simulink model "BLAC0_ControlloCoppiaCompensazioneFCEM"  (R2018b)
settings: Solver=VariableStepAuto  StartTime=0.0  StopTime=0.1  RelTol=1e-3
values from neighbouring files (symbols this model uses):
  B = 3.8e-005    (= 3.8e-05)    [BLAC0_v1.m]    (also in BLAC1_v1.m = 0; BLAC1_v2.m = 0; CAE_11_v_1.m = 0; CAE_14_v1.M = 0)
  Crn = 0.6    [BLAC0_v1.m]    (also in BLAC1_v1.m; BLAC1_v2.m; CAE_11_v_1.m; CAE_14_v1.M)
  J = 0.0000251    (= 2.51e-05)    [BLAC0_v1.m]    (also in BLAC1_v1.m = 0.001; BLAC1_v2.m = 0.001; CAE_11_v_1.m = 0.001; CAE_14_v1.M = 0.001)
  Kc = ms*np*lambdaf/2    (= 0.27)    [BLAC0_v1.m]    (also in BLAC1_v1.m = 0.6; BLAC1_v2.m = 0.6; CAE_11_v_1.m = 0.6; CAE_14_v1.M = 0.6)
  Lsd = 0.005/2    (= 0.0025)    [BLAC0_v1.m]    (also in BLAC1_v1.m = 0.005; BLAC1_v2.m = 0.005; CAE_11_v_1.m = 0.005; CAE_14_v1.M = 0.005)
  Lsq = Lsd    (= 0.0025)    [BLAC0_v1.m]    (also in BLAC1_v1.m = 0.005; BLAC1_v2.m = 0.005; CAE_11_v_1.m = 0.005; CAE_14_v1.M = 0.005)
  np = 2    [BLAC0_v1.m]    (also in BLAC1_v1.m = 4; BLAC1_v2.m = 4; CAE_11_v_1.m = 4; CAE_14_v1.M = 4)
  PSIPM = lambdaf    (= 0.09)    [BLAC0_v1.m]
  Rs = 3.1/2    (= 1.55)    [BLAC0_v1.m]    (also in BLAC1_v1.m = 1; BLAC1_v2.m = 1; CAE_11_v_1.m = 1; CAE_14_v1.M = 1)
  wrr = 1256.6    [BLAC0_v1.m]    (also in BLAC1_v1.m = 300; BLAC1_v2.m = 300)
settings Model: Creator=anton  LastModifiedBy=anton

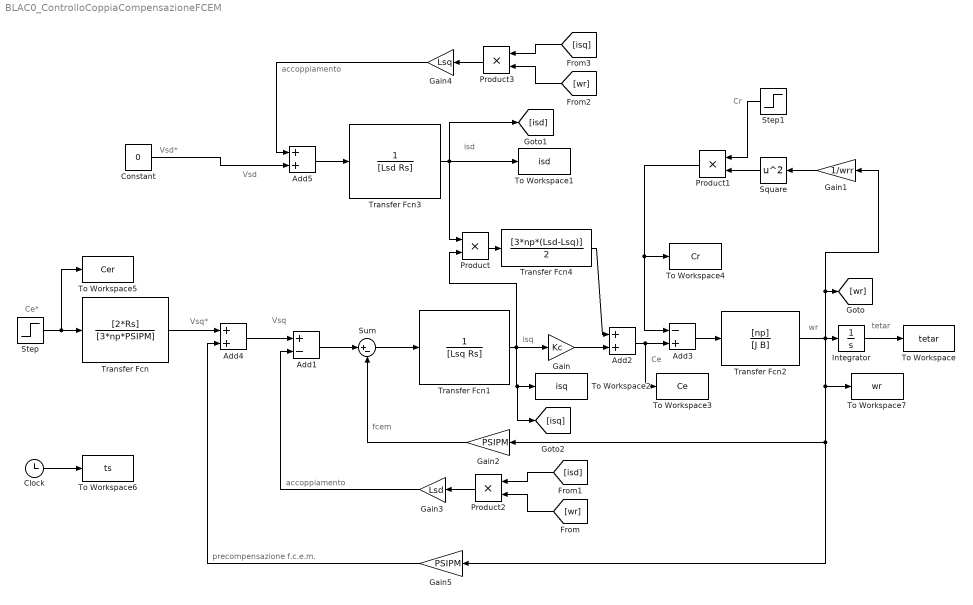
== system BLAC0_ControlloCoppiaCompensazioneFCEM ==
  note: precompensazione f.c.e.m.
  note: accoppiamento
  note: accoppiamento
  note: fcem
  note: Cr
  note: isd
  note: Vsd
  note: Vsd*
  note: tetar
  note: wr
  note: Ce
  note: isq
  note: Vsq
  note: Vsq*
  note: Ce*
  Add1 : Sum  Inputs=+-
  Add2 : Sum
  Add3 : Sum  Inputs=-+
  Add4 : Sum
  Add5 : Sum
  Clock : Clock
  Constant : Constant  Value=0
  Gain : Gain  Gain=Kc
  Gain1 : Gain  Gain=1/wrr
  Gain2 : Gain  Gain=PSIPM
  Gain3 : Gain  Gain=Lsd
  Gain4 : Gain  Gain=Lsq
  Gain5 : Gain  Gain=PSIPM
  Integrator : Integrator
  Product{,1..3} (4 alike) : Product
  Square : Math  Operator=square  SaturateOnIntegerOverflow=on
  Step : Step  Time=0  After=Crn  SampleTime=0
  Step1 : Step  Time=0  After=Crn  SampleTime=0
  Sum : Sum  Inputs=|+-
  To Workspace : ToWorkspace  VariableName=tetar  SampleTime=-1
  To Workspace1 : ToWorkspace  VariableName=isd  SampleTime=-1
  To Workspace2 : ToWorkspace  VariableName=isq  SampleTime=-1
  To Workspace3 : ToWorkspace  VariableName=Ce  SampleTime=-1
  To Workspace4 : ToWorkspace  VariableName=Cr  SampleTime=-1
  To Workspace5 : ToWorkspace  VariableName=Cer  SampleTime=-1
  To Workspace6 : ToWorkspace  VariableName=ts  SampleTime=-1
  To Workspace7 : ToWorkspace  VariableName=wr  SampleTime=-1
  Transfer Fcn : TransferFcn  Numerator=[2*Rs]  Denominator=[3*np*PSIPM]
  Transfer Fcn1 : TransferFcn  Denominator=[Lsq Rs]
  Transfer Fcn2 : TransferFcn  Numerator=[np]  Denominator=[J B]
  Transfer Fcn3 : TransferFcn  Denominator=[Lsd Rs]
  Transfer Fcn4 : TransferFcn  Numerator=[3*np*(Lsd-Lsq)]  Denominator=[2]
  wires:
  Step/1 -> To Workspace5/1, Transfer Fcn/1
  Add1/1 -> Sum/1
  Sum/1 -> Transfer Fcn1/1
  Transfer Fcn1/1 -> Gain/1, [isq], To Workspace2/1, Product/2
  Gain/1 -> Add2/2
  Add2/1 -> To Workspace3/1, Add3/2
  Add3/1 -> Transfer Fcn2/1
  Transfer Fcn2/1 -> To Workspace7/1, Gain5/1, Gain2/1, [wr], Gain1/1, Integrator/1
  Integrator/1 -> To Workspace/1
  Constant/1 -> Add5/2
  Add5/1 -> Transfer Fcn3/1
  Transfer Fcn3/1 -> [isd], To Workspace1/1, Product/1
  Product/1 -> Transfer Fcn4/1
  Transfer Fcn4/1 -> Add2/1
  Step1/1 -> Product1/1
  Product1/1 -> To Workspace4/1, Add3/1
  Square/1 -> Product1/2
  Gain1/1 -> Square/1
  Gain2/1 -> Sum/2
  Gain3/1 -> Add1/2
  Product2/1 -> Gain3/1
  [wr] -> Product2/2
  [isd] -> Product2/1
  [wr] -> Product3/2
  [isq] -> Product3/1
  Product3/1 -> Gain4/1
  Gain4/1 -> Add5/1
  Clock/1 -> To Workspace6/1
  Transfer Fcn/1 -> Add4/1
  Add4/1 -> Add1/1
  Gain5/1 -> Add4/2
